simulink model "LoadFlow58BusNetwork_2024"  (R2024a)
settings: Solver=FixedStepDiscrete  StartTime=0.0  StopTime=4.5  FixedStep=75e-6  RelTol=1e-3  EnableMultiTasking=on
undefined symbols (not defined in the file): D1, D11, Delta
libraries: spsSeriesRLCBranchLib x41, spsLoadFlowBusLib x29, spsDistributedParametersLineLib x19, spsThreePhaseSeriesRLCLoadLib x15, spsThreePhaseTransformerTwoWindingsLib x13, spsThreePhaseParallelRLCLoadLib x11, spsThreePhaseVIMeasurementLib x11, spsSynchronousMachinepuStandardLib x7, spsExcitationSystemLib x7, spsHydraulicTurbineandGovernorLib x7, spsGenericPowerSystemStabilizerLib x7, spsMultiBandPowerSystemStabilizerLib x7
(part 3 of 5)

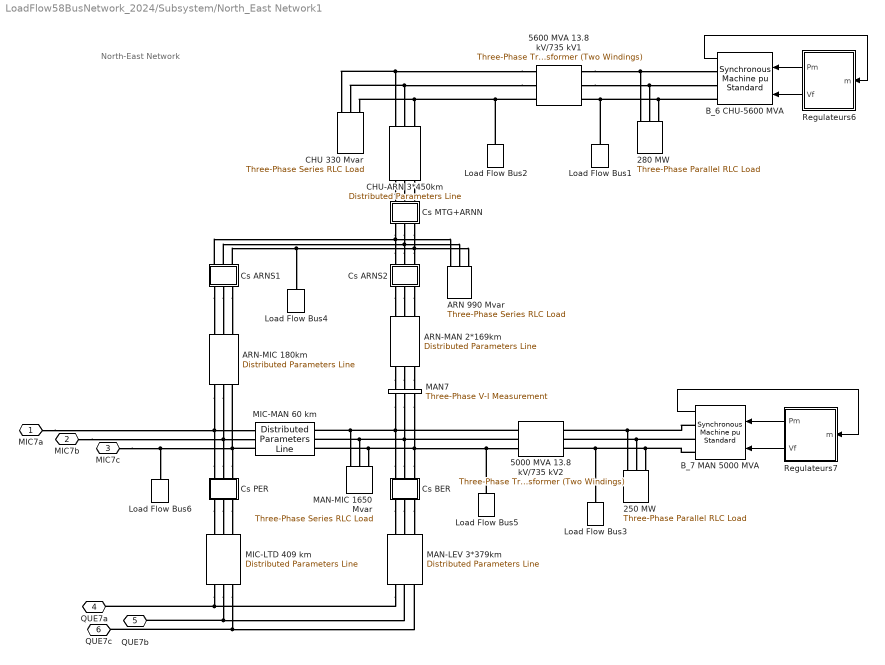
== system LoadFlow58BusNetwork_2024/Subsystem/North_East Network1 ==
  note: North-East Network
  250 MW : spsThreePhaseParallelRLCLoadLib/Three-Phase Parallel RLC Load  LConnTagsString=A|B|C  Configuration=Y (grounded)  NominalVoltage=(13800)*1  Vabc=[1e3 1e3 1e3]  Vabcp=[1e3 1e3 1e3]  NominalFrequency=60  UnbalancedPower=off  ActivePower=250000000  InductivePower=0  CapacitivePower=0  Pabc=[10e3 9e3 11e3]  QLabc=[100 90 110]  QCabc=[100 90 110]  Pabcp=[10e3 9e3 11e3]  QLabcp=[100 90 110]  QCabcp=[100 90 110]  Measurements=None  LoadType=constant PQ
  280 MW : spsThreePhaseParallelRLCLoadLib/Three-Phase Parallel RLC Load  LConnTagsString=A|B|C  Configuration=Y (grounded)  NominalVoltage=(13800)*1  Vabc=[1e3 1e3 1e3]  Vabcp=[1e3 1e3 1e3]  NominalFrequency=60  UnbalancedPower=off  ActivePower=280000000  InductivePower=0  CapacitivePower=0  Pabc=[10e3 9e3 11e3]  QLabc=[100 90 110]  QCabc=[100 90 110]  Pabcp=[10e3 9e3 11e3]  QLabcp=[100 90 110]  QCabcp=[100 90 110]  Measurements=None  LoadType=constant PQ
  5000 MVA 13.8 kV/735 kV2 : spsThreePhaseTransformerTwoWindingsLib/Three-Phase Transformer (Two Windings)  Winding1Connection=Delta (D1)  Winding2Connection=Yg  CoreType=Three single-phase transformers  SetSaturation=off  Hysteresis=off  DataFile='basic_model'  SetInitialFlux=off  Measurements=None  UNITS=pu  NominalPower=[ 5000e6 60 ]  Winding1="[ 13.8e3 0.002  0.0]"  Winding2=[ 735e3 0.002 0.12]  Rm=500  Lm=500  L0=0.5  Saturation="[ 0,0  ;  0.005,1.2  ;  1.0,1.4 ]"  InitialFluxes=[ 0.8 , -0.8 , 0.7 ]  BreakLoop=off  DiscreteSolver=Trapezoidal iterative  DataType=off  TransfoNumber=0
  5600 MVA 13.8 kV/735 kV1 : spsThreePhaseTransformerTwoWindingsLib/Three-Phase Transformer (Two Windings)  Winding1Connection=Delta (D1)  Winding2Connection=Yg  CoreType=Three single-phase transformers  SetSaturation=off  Hysteresis=off  DataFile='basic_model'  SetInitialFlux=off  Measurements=None  UNITS=pu  NominalPower=[ 5600e6 60 ]  Winding1="[ 13.8e3 0.002  0.0]"  Winding2=[ 735e3 0.002 0.12]  Rm=500  Lm=500  L0=0.5  Saturation="[ 0,0  ;  0.005,1.2  ;  1.0,1.4 ]"  InitialFluxes=[ 0.8 , -0.8 , 0.7 ]  BreakLoop=off  DiscreteSolver=Trapezoidal iterative  DataType=off  TransfoNumber=0
  ARN 990 Mvar : spsThreePhaseSeriesRLCLoadLib/Three-Phase Series RLC Load  LConnTagsString=A|B|C  Configuration=Y (grounded)  NominalVoltage=735e3  Vabc=[1e3 1e3 1e3]  Vabcp=[1e3 1e3 1e3]  NominalFrequency=60  UnbalancedPower=off  ActivePower=3300000  InductivePower=990e6  CapacitivePower=0  Pabc=[10e3 9e3 11e3]  QLabc=[100 90 110]  QCabc=[100 90 110]  Pabcp=[10e3 9e3 11e3]  QLabcp=[100 90 110]  QCabcp=[100 90 110]  Measurements=None  LoadType=constant Z
  ARN-MAN 2*169km : spsDistributedParametersLineLib/Distributed Parameters Line  Phases=3  Length=169  Frequency=60  Resistance="[0.01273  0.3864]/2"  Inductance="[0.9337e-3  4.1264e-3]/2"  Capacitance=[12.74e-9 7.751e-9]*2  x1=[-0.000975 1.60994599123016e-09 347873.977312517 -681165.145140754;-0.0009 1.53689774042001e-09 366991.883229411 -671058.367402052;-0.000825 1.46262091707149e-09 385816.421450015 -660415.155871986;-0.00075 1.38717489694071e-09 404332.543926502 -649244.018571007;-0.000675 1.31061999042181e-09 422525.449153869 -637553.885535348;-0.0006 1.23301739433572e-09 440380.594002039 -625354.101678494;-0.000525 1.1544291430104e-09 457883.705341412 -612654.419320997;-0.00045 1.07491805869151e-09 475020.791452591 -599464.990394622;-0.000375 9.94547701323305e-10 491778.153211145 -585796.358327047;-0.0003 9.13382317739751e-10 508142.39503848 -571659.449613611;-0.000225 8.31486790306614e-10 524100.43561006 -557065.565082836;-0.00015 7.4892658505548e-10 539639.51831242 -542026.370862723;-7.5e-05 6.65767699351214e-10 554747.221440602 -526553.889055024]  x2=[-0.000975 1.45072483719961e-09 232985.418240267 -689450.364518849;-0.0009 1.40774718437802e-09 252383.458947605 -682588.200672037;-0.000825 1.36364419999649e-09 271579.748179457 -675180.386261559;-0.00075 1.31845113930594e-09 290558.940715924 -667232.842980908;-0.000675 1.2722041289476e-09 309305.864880883 -658751.923974585;-0.0006 1.22494013807397e-09 327805.534669995 -649744.408759478;-0.000525 1.17669694879617e-09 346043.161730285 -640217.497805431;-0.00045 1.12751312598156e-09 364004.167181725 -630178.806779295;-0.000375 1.07742798642558e-09 381674.193271371 -619636.360457079;-0.0003 1.02648156742245e-09 399039.114850727 -608598.586309068;-0.000225 9.7471459476002e-10 416085.050667174 -597074.307763032;-0.00015 9.2216845016417e-10 432798.374460433 -585072.737150913;-7.5e-05 8.68885138218909e-10 449165.725855185 -572603.468344629]  x3=[-0.000975 -3.46324088240297e-12 1583.75858462542 -1421.24992657593;-0.0009 -3.61811610296408e-12 1623.30400424489 -1375.90902523653;-0.000825 -3.7700990568715e-12 1661.55177948074 -1329.46824327446;-0.00075 -3.91906825127732e-12 1698.47133564667 -1281.96470474027;-0.000675 -4.06490460248682e-12 1734.03315981437 -1233.43638323582;-0.0006 -4.20749153115222e-12 1768.20882440571 -1183.92207155882;-0.000525 -4.34671505546439e-12 1800.97100991732 -1133.46135069244;-0.00045 -4.4824638822682e-12 1832.29352675939 -1082.09455816485;-0.000375 -4.61462949602852e-12 1862.15133619119 -1029.86275580407;-0.0003 -4.74310624557591e-12 1890.52057033672 -976.807696913729;-0.000225 -4.86779142856255e-12 1917.37855126425 -922.971792896131;-0.00015 -4.9885853735609e-12 1942.70380911478 -868.398079349235;-7.5e-05 -5.10539151973954e-12 1966.47609926466 -813.130181664643]  x4=[-0.000975 1.11781487123881e-11 1569.30174481155 -9115.59279820464;-0.0009 1.10714227902124e-11 1826.37892658973 -9067.58416140609;-0.000825 1.09558465420566e-11 2081.99612899853 -9012.3270365676;-0.00075 1.08315123578052e-11 2335.94901555742 -8949.86559538931;-0.000675 1.06985196283027e-11 2588.03458021449 -8880.2497685916;-0.0006 1.05569746659022e-11 2838.0513096264 -8803.53520600126;-0.000525 1.04069906194808e-11 3085.79934424503 -8719.78323206585;-0.00045 1.02486873839906e-11 3331.08063808218 -8629.06079683187;-0.000375 1.00821915046157e-11 3573.6991170245 -8531.44042242597;-0.0003 9.90763607561482e-12 3813.46083557209 -8427.0001450818;-0.000225 9.72516063392696e-12 4050.17413187564 -8315.82345275907;-0.00015 9.53491104762829e-12 4283.64978094791 -8197.99921840458;-7.5e-05 9.33703939932717e-12 4513.70114592732 -8073.62162890849]  x5=0.000955765248222805  V1=ones(3,3)  V2=ones(3,3)  I1=ones(3,3)  I2=ones(3,3)  nHarmo=1  Measurements=None  Decoupling=on  VsMag0=[624500.542746141 624501.904306222 624500.043261921]  VrMag0=[594207.380493472 594208.10130569 594207.286862311]  VsAngle0=[18.1135948354222 -101.886530201489 138.113424134252]  VrAngle0=[9.73160889879769 -110.268441654031 129.731523430554]  IsMag0=[1744.35611857441 1744.39210598369 1744.37536737747]  IrMag0=[7582.44376493555 7582.43378992705 7582.40838117062]  IsAngle0=[39.1559168024775 -80.8440356055341 159.154916919463]  IrAngle0=[0.828149284034121 -119.172115933986 120.828081951988]
      settings: AttributesFormatString=\n  LibrarySourceBlock=sps_lib/Power Grid Elements/Distributed Parameters Line
  ARN-MIC 180km : spsDistributedParametersLineLib/Distributed Parameters Line  Phases=3  Length=180  Frequency=60  Resistance="[0.01273  0.3864]"  Inductance="[0.9337e-3  4.1264e-3]"  Capacitance=[12.74e-9 7.751e-9]  x1=[-0.00105 1.19354121063199e-09 336203.730988114 -674396.627297907;-0.000975 1.12512510468791e-09 355134.952563332 -664622.476598179;-0.0009 1.05580959095014e-09 373782.284691218 -654317.036859723;-0.000825 9.85650079179792e-10 392130.820979783 -643488.546093388;-0.00075 9.14702653817098e-10 410165.893889859 -632145.660429011;-0.000675 8.43024029148362e-10 427873.086460108 -620297.44719584;-0.0006 7.70671503969425e-10 445238.243831719 -607953.37767425;-0.000525 6.97702915781885e-10 462247.484563584 -595123.319524545;-0.00045 6.24176594558681e-10 478887.211728913 -581817.528898905;-0.000375 5.5015131611601e-10 495144.123784406 -568046.64224277;-0.0003 4.75686255128832e-10 511005.225203304 -553821.667792231;-0.000225 4.00840937827548e-10 526457.836863818 -539153.976774214;-0.00015 3.25675194413637e-10 541489.606184617 -524055.294316497;-7.5e-05 2.50249111232309e-10 556088.516999301 -508537.690074818]  x2=[-0.00105 4.52654920431781e-09 192165.578486817 -719334.039084965;-0.000975 4.47031749550698e-09 212424.764832674 -713613.931123342;-0.0009 4.41051228328839e-09 232514.142071731 -707323.371103839;-0.000825 4.34718137503364e-09 252417.651063202 -700467.387603885;-0.00075 4.2803753965018e-09 272119.381246533 -693051.461191792;-0.000675 4.21014775136993e-09 291603.583360062 -685081.520045664;-0.0006 4.13655457854304e-09 310854.682030736 -676563.935214511;-0.000525 4.05965470727746e-09 329857.288224832 -667505.515525323;-0.00045 3.97950961015369e-09 348596.211549706 -657913.502140201;-0.000375 3.8961833539361e-09 367056.472396769 -647795.562767882;-0.0003 3.80974254835898e-09 385223.31391595 -637159.785534291;-0.000225 3.72025629287972e-09 403082.213812101 -626014.672517016;-0.00015 3.62779612144176e-09 420618.895953895 -614369.132948876;-7.5e-05 3.53243594529146e-09 437819.341785948 -602232.476096019]  x3=[-0.00105 3.53596874152127e-12 149.00166074942 -364.540935538888;-0.000975 3.79801966073249e-12 159.247423691846 -360.18329187299;-0.0009 4.05703450113857e-12 169.365886680341 -355.537723194559;-0.000825 4.31280621023915e-12 179.348961170408 -350.607943100115;-0.00075 4.56513032804341e-12 189.188666845046 -345.397892380438;-0.000675 4.81380515051227e-12 198.877137994092 -339.911735870358;-0.0006 5.05863189079749e-12 208.406629801948 -334.153859119447;-0.000525 5.29941483814888e-12 217.769524538669 -328.128864886281;-0.00045 5.53596151436242e-12 226.958337649459 -321.841569459065;-0.000375 5.76808282764443e-12 235.96572373771 -315.296998805564;-0.0003 5.99559322376864e-12 244.784482436803 -308.500384555424;-0.000225 6.21831083440543e-12 253.407564165964 -301.457159818085;-0.00015 6.43605762250454e-12 261.828075765596 -294.172954839637;-7.5e-05 6.6486595246152e-12 270.039286007565 -286.653592502086]  x4=[-0.00105 4.83329412277315e-12 1187.65933351918 -4979.46515427106;-0.000975 4.45670929323629e-12 1327.95758028639 -4943.89904376734;-0.0009 4.07656183848036e-12 1467.19427808235 -4904.38085601222;-0.000825 3.69315564256423e-12 1605.25812322123 -4860.94218124035;-0.00075 3.30679719453461e-12 1742.03874957769 -4813.61774366371;-0.000675 2.91779534342338e-12 1877.42681681182 -4762.4453737136;-0.0006 2.52646105135838e-12 2011.31409777419 -4707.46597779961;-0.000525 2.13310714498507e-12 2143.59356502093 -4648.7235056096;-0.00045 1.7380480653977e-12 2274.15947636987 -4586.26491497707;-0.000375 1.34159961677987e-12 2402.90745942922 -4520.14013434371;-0.0003 9.44078713955551e-13 2529.73459503121 -4450.40202284742;-0.000225 5.45803129052187e-13 2654.53949950417 -4377.1063280675;-0.00015 1.47091237478525e-13 2777.22240571704 -4300.31164146089;-7.5e-05 -2.51738236579805e-13 2897.68524283171 -4220.07935152508]  x5=0.00101797482059234  V1=ones(3,3)  V2=ones(3,3)  I1=ones(3,3)  I2=ones(3,3)  nHarmo=1  Measurements=None  Decoupling=on  VsMag0=[615273.936100311 615275.237959029 615273.425867059]  VrMag0=[607930.23167611 607930.976808519 607930.152146887]  VsAngle0=[19.1774103741909 -100.822714483793 139.177242954885]  VrAngle0=[7.63692875074935 -112.363120449623 127.636843332422]  IsMag0=[322.896150602406 322.910343515381 322.909058922126]  IrMag0=[4197.50413399086 4197.49907033608 4197.48826872802]  IsAngle0=[14.9112658694316 -105.087543385488 134.909680310748]  IrAngle0=[6.09512812442721 -113.905082032175 126.09508290497]
      settings: AttributesFormatString=\n  LibrarySourceBlock=sps_lib/Power Grid Elements/Distributed Parameters Line
  "B_6 CHU-5600 MVA " : spsSynchronousMachinepuStandardLib/Synchronous Machine pu Standard  PresetModel=No  MechanicalLoad=Mechanical power Pm  ShowDetailedParameters=on  RotorType=Salient-pole  Units=per unit standard parameters  MeasurementBus=off  NominalParameters="[ 5600E6  13800   60 ]"  Reactances1=[ 31 32 33 34 35 36 37 ]  Reactances2=[ 1.305, 0.296, 0.252, 0.474, 0.243, 0.18 ]  dAxisTimeConstants=Short-circuit  qAxisTimeConstants=Open-circuit  TimeConstants1=[]  TimeConstants2=[]  TimeConstants3=[]  TimeConstants4=[]  TimeConstants5=[ 1.01, 0.053, 0.1 ]  TimeConstants6=[]  TimeConstants7=[]  TimeConstants8=[]  StatorResistance=2.8544e-3  Mechanical="[ 4.0 0  32]"  PolePairs=32  InitialConditions=[0 -61.7964 0.894782 0.894782 0.894782 8.48442 -111.516 128.484 1.31361]  SetSaturation=off  Saturation=[0.6404,0.7127,0.8441,0.9214,0.9956,1.082,1.19,1.316,1.457;0.7,0.7698,0.8872,0.9466,0.9969,1.046,1.1,1.151,1.201]  LoadFlowParameters=[1 5000000000 0 0 0]  TsPowergui=0  TsBlock=-1  IterativeModel=Trapezoidal non iterative  IterativeDiscreteModel=Trapezoidal non iterative  BusType=PV  Pref=5000000000  Qref=0  Qmin=-Inf  Qmax=Inf  PLF=0  QLF=0
  B_7 MAN 5000 MVA : spsSynchronousMachinepuStandardLib/Synchronous Machine pu Standard  PresetModel=No  MechanicalLoad=Mechanical power Pm  ShowDetailedParameters=on  RotorType=Salient-pole  Units=per unit standard parameters  MeasurementBus=off  NominalParameters="[ 5000E6  13800   60 ]"  Reactances1=[ 31 32 33 34 35 36 37 ]  Reactances2=[ 1.305, 0.296, 0.252, 0.474, 0.243, 0.18 ]  dAxisTimeConstants=Short-circuit  qAxisTimeConstants=Open-circuit  TimeConstants1=[]  TimeConstants2=[]  TimeConstants3=[]  TimeConstants4=[]  TimeConstants5=[ 1.01, 0.053, 0.1 ]  TimeConstants6=[]  TimeConstants7=[]  TimeConstants8=[]  StatorResistance=2.8544e-3  Mechanical="[ 3.7 0  32]"  PolePairs=32  InitialConditions=[0 -81.9543 0.907703 0.907703 0.907703 -8.76021 -128.76 111.24 1.25655]  SetSaturation=off  Saturation=[0.6404,0.7127,0.8441,0.9214,0.9956,1.082,1.19,1.316,1.457;0.7,0.7698,0.8872,0.9466,0.9969,1.046,1.1,1.151,1.201]  LoadFlowParameters=[1 4500000000 0 0 0]  TsPowergui=0  TsBlock=-1  IterativeModel=Trapezoidal non iterative  IterativeDiscreteModel=Trapezoidal non iterative  BusType=PV  Pref=4500000000  Qref=0  Qmin=-Inf  Qmax=Inf  PLF=0  QLF=0
  CHU 330 Mvar : spsThreePhaseSeriesRLCLoadLib/Three-Phase Series RLC Load  LConnTagsString=A|B|C  Configuration=Y (grounded)  NominalVoltage=735e3  Vabc=[1e3 1e3 1e3]  Vabcp=[1e3 1e3 1e3]  NominalFrequency=60  UnbalancedPower=off  ActivePower=1100000  InductivePower=330e6  CapacitivePower=0  Pabc=[10e3 9e3 11e3]  QLabc=[100 90 110]  QCabc=[100 90 110]  Pabcp=[10e3 9e3 11e3]  QLabcp=[100 90 110]  QCabcp=[100 90 110]  Measurements=None  LoadType=constant Z
  CHU-ARN 3*450km : spsDistributedParametersLineLib/Distributed Parameters Line  Phases=3  Length=450  Frequency=60  Resistance="[0.01273  0.3864]/3"  Inductance="[0.9337e-3  4.1264e-3]/3"  Capacitance=[12.74e-9 7.751e-9]*3  x1=[-0.00255 1.80867377993606e-09 0 0;-0.002475 1.72308488593625e-09 0 0;-0.0024 1.6361185842427e-09 0 0;-0.002325 1.54784439438636e-09 0 0;-0.00225 1.45833288140396e-09 0 0;-0.002175 1.36765559942941e-09 0 0;-0.0021 1.2758850344945e-09 0 0;-0.002025 1.18309454658472e-09 0 0;-0.00195 1.08935831099635e-09 0 0;-0.001875 9.94751259041912e-10 0 0;-0.0018 8.993490181512e-10 0 0;-0.001725 8.03227851415879e-10 0 0;-0.00165 7.06464596625934e-10 0 0;-0.001575 6.09136604846718e-10 336692.129653521 -649852.524072729;-0.0015 5.1132167858569e-10 354929.318551966 -640074.408280399;-0.001425 4.13098009598284e-10 372882.782383762 -629784.626799556;-0.00135 3.14544116382617e-10 390538.169424619 -618991.405124078;-0.001275 2.15738781413e-10 407881.366228272 -607703.37119023;-0.0012 1.16760988162435e-10 424898.508908555 -595929.548479625;-0.001125 1.76898579644369e-11 441575.994221983 -583679.348805994;-0.00105 -8.13954132353542e-11 457900.490441969 -570962.564791521;-0.000975 -1.80415618187197e-10 473858.948016008 -557789.362038774;-0.0009 -2.79291601654312e-10 489438.609997288 -544170.271004476;-0.000825 -3.7794432368837e-10 504627.022242398 -530116.178581621;-0.00075 -4.76294922812813e-10 519412.04336698 -515638.319396658;-0.000675 -5.74264779063516e-10 533781.854451365 -500748.266828701;-0.0006 -6.71775576836382e-10 547724.968488438 -485457.923757945;-0.000525 -7.68749367491635e-10 561230.239566175 -469779.513050693;-0.00045 -8.65108631664776e-10 574286.871777512 -453725.567788576;-0.000375 -9.60776341234369e-10 586884.427850435 -437308.921249803;-0.0003 -1.05567602089715e-09 599012.837491367 -420542.696650433;-0.000225 -1.14973180930121e-09 610662.405435212 -403440.29665388;-0.00015 -1.24286851968841e-09 621823.8191956 -386015.392657025;-7.5e-05 -1.33501169999749e-09 632488.156509147 -368281.913861514]  x2=[-0.00255 2.59530396061635e-09 0 0;-0.002475 2.56712725861336e-09 0 0;-0.0024 2.53689843435821e-09 0 0;-0.002325 2.50464165231048e-09 0 0;-0.00225 2.47038269804819e-09 0 0;-0.002175 2.43414895765521e-09 0 0;-0.0021 2.39596939582921e-09 0 0;-0.002025 2.35587453272774e-09 0 0;-0.00195 2.3138964195709e-09 0 0;-0.001875 2.27006861302005e-09 0 0;-0.0018 2.22442614835317e-09 0 0;-0.001725 2.17700551145816e-09 0 0;-0.00165 2.12784460966659e-09 0 0;-0.001575 2.07698274145117e-09 24661.2186379731 -733238.396736884;-0.0015 2.02446056501113e-09 45380.4401577959 -732248.159297742;-0.001425 1.97032006577071e-09 66063.3852481006 -730672.57388383;-0.00135 1.91460452281662e-09 86693.5202790416 -728512.899994021;-0.001275 1.85735847430142e-09 107254.353836327 -725770.864038578;-0.0012 1.79862768184041e-09 127729.449904202 -722448.657959089;-0.001125 1.73845909393045e-09 148102.44100415 -718548.937476262;-0.00105 1.67690080842013e-09 168357.041278802 -714074.819966984;-0.000975 1.61400203406099e-09 188477.059510606 -709029.881972336;-0.0009 1.54981305117089e-09 208446.412064832 -703418.15633856;-0.000825 1.48438517144061e-09 228249.135746591 -697244.128993266;-0.00075 1.41777069691614e-09 247869.400561563 -690512.735359448;-0.000675 1.35002287818918e-09 267291.522370255 -683229.356410182;-0.0006 1.28119587182943e-09 286499.975425661 -675399.814367161;-0.000525 1.2113446970927e-09 305479.404784309 -667030.3680465;-0.00045 1.1405251919393e-09 324214.638580764 -658127.707855528;-0.000375 1.06879396839809e-09 342690.700155788 -648698.950444589;-0.0003 9.96208367311644e-10 360892.82002845 -638751.633018091;-0.000225 9.22826412498863e-10 378806.447702628 -628293.707309386;-0.00015 8.48706764371648e-10 396417.263298445 -617333.533224274;-7.5e-05 7.73908673042644e-10 413711.188999368 -605879.872158222]  x3=[-0.00255 4.24136020094849e-12 0 0;-0.002475 4.2220551602755e-12 0 0;-0.0024 4.199375073307e-12 0 0;-0.002325 4.17333807015748e-12 0 0;-0.00225 4.1439649644089e-12 0 0;-0.002175 4.11127923647256e-12 0 0;-0.0021 4.07530701481927e-12 0 0;-0.002025 4.03607705509262e-12 0 0;-0.00195 3.99362071712217e-12 0 0;-0.001875 3.94797193985491e-12 0 0;-0.0018 3.89916721422492e-12 0 0;-0.001725 3.84724555398313e-12 0 0;-0.00165 3.79224846451033e-12 0 0;-0.001575 3.73421990963834e-12 -336.540930618498 -2064.60581280805;-0.0015 3.67320627650607e-12 -278.039507495715 -2073.29664773843;-0.001425 3.6092563384783e-12 -219.315823844787 -2080.33012105111;-0.00135 3.54242121615703e-12 -160.416822479922 -2085.70061029514;-0.001275 3.47275433651642e-12 -101.389586361627 -2089.40382238359;-0.0012 3.40031139019412e-12 -42.2813009593069 -2091.43679702537;-0.001125 3.32515028697301e-12 16.8607834680746 -2091.79790909167;-0.00105 3.247331109489e-12 75.9893896431304 -2090.48686991503;-0.000975 3.16691606520189e-12 135.057251062782 -2087.50472752009;-0.0009 3.08396943666771e-12 194.017149782379 -2082.85386578587;-0.000825 2.99855753015217e-12 252.821954161003 -2076.53800254008;-0.00075 2.91074862262649e-12 311.424656537775 -2068.56218658714;-0.000675 2.82061290718783e-12 369.778410809068 -2058.93279367232;-0.0006 2.72822243694799e-12 427.83656987656 -2047.65752138496;-0.000525 2.63365106743526e-12 485.552722936212 -2034.74538300522;-0.00045 2.53697439755543e-12 542.880732578354 -2020.20670029895;-0.000375 2.43826970915921e-12 599.774771669227 -2004.05309526666;-0.0003 2.33761590526426e-12 656.189359984489 -1986.29748085305;-0.000225 2.23509344698136e-12 712.079400565414 -1966.95405062462;-0.00015 2.13078428919503e-12 767.400215768706 -1946.03826742353;-7.5e-05 2.02477181505001e-12 822.10758298113 -1923.56685100685]  x4=[-0.00255 1.92507826273785e-11 0 0;-0.002475 1.90857971627026e-11 0 0;-0.0024 1.89055548037973e-11 0 0;-0.002325 1.87101996336465e-11 0 0;-0.00225 1.84998878161842e-11 0 0;-0.002175 1.82747874714595e-11 0 0;-0.0021 1.80350785412437e-11 0 0;-0.002025 1.7780952645188e-11 0 0;-0.00195 1.75126129276454e-11 0 0;-0.001875 1.72302738952804e-11 0 0;-0.0018 1.69341612455956e-11 0 0;-0.001725 1.66245116865124e-11 0 0;-0.00165 1.63015727471505e-11 0 0;-0.001575 1.5965602579957e-11 -291.74302430487 -14207.2379327614;-0.0015 1.5616869754343e-11 110.022151991721 -14209.8063832457;-0.001425 1.52556530419935e-11 511.699378263407 -14201.0157319245;-0.00135 1.48822411940216e-11 912.967559881373 -14180.8730059101;-0.001275 1.44969327101451e-11 1313.50592920084 -14149.3943069894;-0.0012 1.41000356000706e-11 1712.99430197782 -14106.6047987527;-0.001125 1.36918671372751e-11 2111.11333331949 -14052.5386864782;-0.00105 1.32727536053828e-11 2507.54477296362 -13987.2391897887;-0.000975 1.28430300373382e-11 2901.97171968297 -13910.7585081029;-0.0009 1.24030399475867e-11 3294.07887461125 -13823.1577789074;-0.000825 1.1953135057474e-11 3683.55279328827 -13724.5070288849;-0.00075 1.14936750140855e-11 4070.08213622259 -13614.8851179355;-0.000675 1.10250271027498e-11 4453.35791777155 -13494.3796761375;-0.0006 1.05475659534367e-11 4833.0737531397 -13363.0870336974;-0.000525 1.00616732412837e-11 5208.92610329811 -13221.1121439446;-0.00045 9.56773738149033e-12 5580.61451762878 -13068.5684994337;-0.000375 9.06615321882548e-12 5947.84187410032 -12905.5780412202;-0.0003 8.55732171199431e-12 6310.31461678274 -12732.2710613825;-0.000225 8.04164961311797e-12 6667.74299051156 -12548.7860988686;-0.00015 7.51954914258228e-12 7019.84127251364 -12355.2698287502;-7.5e-05 6.99143765951497e-12 7366.32800080966 -12151.8769449726]  x5=0.00254493705148084  V1=ones(3,3)  V2=ones(3,3)  I1=ones(3,3)  I2=ones(3,3)  nHarmo=1  Measurements=None  Decoupling=on  VsMag0=[597589.636778606 597591.191030923 597588.179734111]  VrMag0=[599025.218159244 599025.681050624 599025.14641932]  VsAngle0=[31.4089201475954 -88.5913271983218 151.408667420084]  VrAngle0=[5.94632207994268 -114.053711405456 125.94626699413]  IsMag0=[1726.1254830947 1726.16866029042 1726.16794416601]  IrMag0=[11726.0675753704 11726.0492062867 11726.0164561755]  IsAngle0=[-5.23898774451376 -125.238187761859 114.760171100737]  IrAngle0=[2.8437567880639 -117.156479810909 122.843716218955]
      settings: AttributesFormatString=\n  LibrarySourceBlock=sps_lib/Power Grid Elements/Distributed Parameters Line
  "Cs ARNS1 " : Subsystem  mask{Xc=25}
      mask prompts: Xc "Condensator Reactance at  60Hz  (ohm):"
      mask help: Series Compensation
      mask init:
      | Cs=1/Xc/(2*pi*60);
      mask Display: disp('Cs')
  Cs ARNS2 : Subsystem  mask{Xc=25/2}
      mask prompts: Xc "Condensator Reactance at  60Hz  (ohm):"
      mask help: Series Compensation
      mask init:
      | Cs=1/Xc/(2*pi*60);
      mask Display: disp('Cs')
  Cs BER : Subsystem  mask{Xc=22/3}
      mask prompts: Xc "Condensator Reactance at  60Hz  (ohm):"
      mask help: Series Compensation
      mask init:
      | Cs=1/Xc/(2*pi*60);
      mask Display: disp('Cs')
  "Cs MTG+ARNN " : Subsystem  mask{Xc=(30+25)/3}
      mask prompts: Xc "Condensator Reactance at  60Hz  (ohm):"
      mask help: Series Compensation
      mask init:
      | Cs=1/Xc/(2*pi*60);
      mask Display: disp('Cs')
  "Cs PER " : Subsystem  mask{Xc=22}
      mask prompts: Xc "Condensator Reactance at  60Hz  (ohm):"
      mask help: Series Compensation
      mask init:
      | Cs=1/Xc/(2*pi*60);
      mask Display: disp('Cs')
  Load Flow Bus1 : spsLoadFlowBusLib/Load Flow Bus  LConnTagsString=a  Phases=single  Connectors=on one side  ID=CHU_13.8  Vbase=13.8e3  Vref=1  Vangle=0  VLF=1  VLFb=1  VLFc=1  angleLF=4.726  angleLFb=0  angleLFc=0
      settings: AttributesFormatString=%<ID>\n%<Vbase>V\n%<VLF>pu\n%<angleLF>deg.
  Load Flow Bus2 : spsLoadFlowBusLib/Load Flow Bus  LConnTagsString=a  Phases=single  Connectors=on one side  ID=CHU7  Vbase=735e3  Vref=1  Vangle=0  VLF=1.009  VLFb=1  VLFc=1  angleLF=28.97  angleLFb=0  angleLFc=0
      settings: AttributesFormatString=%<ID>\n%<Vbase>V\n%<VLF>pu\n%<angleLF>deg.
  Load Flow Bus3 : spsLoadFlowBusLib/Load Flow Bus  LConnTagsString=a  Phases=single  Connectors=on one side  ID=MAN_13.8  Vbase=13.8e3  Vref=1  Vangle=0  VLF=1  VLFb=1  VLFc=1  angleLF=-16.23  angleLFb=0  angleLFc=0
      settings: AttributesFormatString=%<ID>\n%<Vbase>V\n%<VLF>pu\n%<angleLF>deg.
  Load Flow Bus4 : spsLoadFlowBusLib/Load Flow Bus  LConnTagsString=a  Phases=single  Connectors=on one side  ID=ARN7  Vbase=735e3  Vref=1  Vangle=0  VLF=1.054  VLFb=1  VLFc=1  angleLF=12.72  angleLFb=0  angleLFc=0
      settings: AttributesFormatString=%<ID>\n%<Vbase>V\n%<VLF>pu\n%<angleLF>deg.
  Load Flow Bus5 : spsLoadFlowBusLib/Load Flow Bus  LConnTagsString=a  Phases=single  Connectors=on one side  ID=MAN7  Vbase=735e3  Vref=1  Vangle=0  VLF=1.016  VLFb=1  VLFc=1  angleLF=7.996  angleLFb=0  angleLFc=0
      settings: AttributesFormatString=%<ID>\n%<Vbase>V\n%<VLF>pu\n%<angleLF>deg.
  Load Flow Bus6 : spsLoadFlowBusLib/Load Flow Bus  LConnTagsString=a  Phases=single  Connectors=on one side  ID=MIC7  Vbase=735e3  Vref=1  Vangle=0  VLF=1.041  VLFb=1  VLFc=1  angleLF=5.981  angleLFb=0  angleLFc=0
      settings: AttributesFormatString=%<ID>\n%<Vbase>V\n%<VLF>pu\n%<angleLF>deg.
  MAN-LEV 3*379km : spsDistributedParametersLineLib/Distributed Parameters Line  Phases=3  Length=379  Frequency=60  Resistance="[0.01273  0.3864]/3"  Inductance="[0.9337e-3  4.1264e-3]/3"  Capacitance=[12.74e-9 7.751e-9]*3  x1=[-0.002175 3.20011367306785e-09 -30838.3336726537 -721772.96842408;-0.0021 3.15830158139619e-09 -10421.0500053442 -722356.328523331;-0.002025 3.11396479176399e-09 10004.5640898923 -722362.248025983;-0.00195 3.06713874632251e-09 30422.1806896704 -721790.722200075;-0.001875 3.01786087709602e-09 50815.47826368 -720642.20791461;-0.0018 2.96617057605919e-09 71168.1547218684 -718917.623274333;-0.001725 2.9121091636478e-09 91463.9404460816 -716618.346885819;-0.00165 2.85571985572775e-09 111686.611295747 -713746.216755433;-0.001575 2.79704772904902e-09 131820.001577206 -710303.528820056;-0.0015 2.73613968521194e-09 151848.016966317 -706293.035111749;-0.001425 2.67304441317485e-09 171754.647374018 -701717.941557819;-0.00135 2.60781235033282e-09 191523.979744542 -696581.905418053;-0.001275 2.5404956421988e-09 211140.210776074 -690889.032361155;-0.0012 2.47114810071929e-09 230587.659553665 -684643.873182745;-0.001125 2.3998251612579e-09 249850.780084318 -677851.420167516;-0.00105 2.32658383828115e-09 268914.173724217 -670517.103098478;-0.000975 2.25148267978202e-09 287762.601488166 -662646.78491648;-0.0009 2.1745817204775e-09 306380.9962314 -654246.757033455;-0.000825 2.09594243381785e-09 324754.474694034 -645323.734303169;-0.00075 2.0156276828456e-09 342868.349398507 -635884.849653465;-0.000675 1.93370166994382e-09 360708.140390532 -625937.648384312;-0.0006 1.85022988551372e-09 378259.58681415 -615490.082136208;-0.000525 1.7652790556226e-09 395508.658311633 -604550.502533759;-0.00045 1.6789170886641e-09 412441.566239148 -593127.654509517;-0.000375 1.5912130210732e-09 429044.774689179 -581230.669313417;-0.0003 1.50223696213964e-09 445305.011310928 -568869.057213396;-0.000225 1.41206003796354e-09 461209.27792003 -556052.699893027;-0.00015 1.32075433459834e-09 476744.860889102 -542791.842552255;-7.5e-05 1.22839284042627e-09 491899.34131082 -529097.08571754]  x2=[-0.002175 1.38351872909083e-08 -379192.175232135 -624794.196144335;-0.0021 1.38990649351923e-08 -361377.32073441 -635264.451513569;-0.002025 1.39518318796298e-08 -343273.586735748 -645226.886200136;-0.00195 1.3993445943133e-08 -324895.445084111 -654673.536386177;-0.001875 1.40238738600562e-08 -306257.586984741 -663596.850564071;-0.0018 1.40430913067881e-08 -287374.911256234 -671989.695572997;-0.001725 1.40510829211958e-08 -268262.512420652 -679845.362301069;-0.00165 1.40478423149052e-08 -248935.668637195 -687157.5710485;-0.001575 1.40333720784072e-08 -229409.829489073 -693920.476547499;-0.0015 1.40076837789875e-08 -209700.603633346 -700128.672634885;-0.001425 1.39707979514796e-08 -189823.746323601 -705777.196573694;-0.00135 1.39227440818497e-08 -169795.146815445 -710861.533020316;-0.001275 1.38635605836259e-08 -149630.815664878 -715377.617633987;-0.0012 1.37932947671911e-08 -129346.871929697 -719321.840325766;-0.001125 1.37120028019639e-08 -108959.530284169 -722691.048144382;-0.00105 1.36197496714975e-08 -88485.0880572684 -725482.547796656;-0.000975 1.35166091215329e-08 -67939.9122048419 -727694.107800476;-0.0009 1.34026636010476e-08 -47340.4262261144 -729323.960268613;-0.000825 1.32780041963472e-08 -26703.0970349947 -730370.802321943;-0.00075 1.31427305582526e-08 -6044.42179667621 -730833.797130944;-0.000675 1.29969508224402e-08 14619.0852599438 -730712.574584651;-0.0006 1.28407815230003e-08 35270.9060434865 -730007.231586512;-0.000525 1.26743474992815e-08 55894.531804401 -728718.331976929;-0.00045 1.24977817960958e-08 76473.4763318061 -726846.906082527;-0.000375 1.23112255573648e-08 96991.2891323149 -724394.449892533;-0.0003 1.21148279132913e-08 117431.568580308 -721362.923862902;-0.000225 1.1908745861147e-08 137777.975029141 -717754.751349158;-0.00015 1.16931441397712e-08 158014.24387281 -713572.816669202;-7.5e-05 1.14681950978812e-08 178124.198547625 -708820.46279763]  x3=[-0.002175 6.58584377734838e-12 -359.273937221319 349.814819581325;-0.0021 8.15999498110593e-12 -369.020063583709 339.517457528038;-0.002025 9.7276232097277e-12 -378.471200953466 328.948690413994;-0.00195 1.12874753251933e-11 -387.619794235985 318.116966749918;-0.001875 1.2838304405588e-11 -396.458530185773 307.030945249974;-0.0018 1.43788707418736e-11 -404.980343252549 295.699487910128;-0.001725 1.59079428288922e-11 -413.178421229337 284.131652924001;-0.00165 1.74242983498131e-11 -421.046210698035 272.336687441887;-0.001575 1.89267251532338e-11 -428.577422268125 260.324020178722;-0.0015 2.04140222221557e-11 -435.766035604308 248.103253876918;-0.001425 2.18850006340581e-11 -442.606304239072 235.684157630072;-0.00135 2.33384845113055e-11 -449.092760166332 223.076659073705;-0.001275 2.47733119611253e-11 -455.220218212464 210.290836449261;-0.0012 2.61883360044078e-11 -460.98378018126 197.336910547718;-0.001125 2.75824254925833e-11 -466.378838769468 184.225236539239;-0.00105 2.89544660118453e-11 -471.401081249799 170.966295695411;-0.000975 3.03033607739956e-11 -476.046492918457 157.570687010676;-0.0009 3.16280314932002e-11 -480.311360304431 144.049118729657;-0.000825 3.29274192479542e-11 -484.192274137989 130.412399787151;-0.00075 3.42004853275678e-11 -487.686132075991 116.671431167632;-0.000675 3.54462120624955e-11 -490.790141181859 102.83719719117;-0.0006 3.66636036378457e-11 -493.501820158208 88.9207567327353;-0.000525 3.78516868894197e-11 -495.819001330353 74.9332343819018;-0.00045 3.90095120816446e-11 -497.73983237912 60.8858115500204;-0.000375 4.01361536667769e-11 -499.262777821557 46.78971753197;-0.0003 4.12307110247718e-11 -500.386620238381 32.6562205296313;-0.000225 4.22923091832245e-11 -501.110461247159 18.4966186442581;-0.00015 4.33200995168102e-11 -501.433722220462 4.32223084494839;-7.5e-05 4.43132604256619e-11 -501.356144748416 -9.85561207956639]  x4=[-0.002175 5.32822560666844e-11 -7842.63207577957 -13937.1348474411;-0.0021 5.25232661185771e-11 -7445.48599612257 -14153.2795346858;-0.002025 5.17222898751674e-11 -7042.38810888003 -14358.1103068229;-0.00195 5.08799676246092e-11 -6633.6606443354 -14551.4634252672;-0.001875 4.99969727064214e-11 -6219.6303329701 -14733.1843264942;-0.0018 4.90740109732314e-11 -5800.62814428016 -14903.1277455959;-0.001725 4.8111820226527e-11 -5376.98902220426 -15061.1578324032;-0.00165 4.7111169626869e-11 -4949.05161737471 -15207.1482600828;-0.001575 4.60728590790364e-11 -4517.15801640526 -15340.9823261204;-0.0015 4.49977185925944e-11 -4081.65346843233 -15462.5530456115;-0.001425 4.38866076183977e-11 -3642.88610912813 -15571.7632367828;-0.00135 4.27404143615584e-11 -3201.20668240631 -15668.5255986787;-0.001275 4.15600550714287e-11 -2756.96826004269 -15752.7627809474;-0.0012 4.03464733091651e-11 -2310.52595943501 -15824.4074456744;-0.001125 3.910063919346e-11 -1862.2366597276 -15883.4023212109;-0.00105 3.78235486250434e-11 -1412.45871652758 -15929.700247956;-0.000975 3.65162224905756e-11 -961.551675440905 -15963.2642160555;-0.0009 3.51797058465658e-11 -509.875984657118 -15984.0673949868;-0.000825 3.38150670839699e-11 -57.7927068125609 -15992.093155007;-0.00075 3.24233970741348e-11 394.336769637563 -15987.3350804463;-0.000675 3.10058082967734e-11 846.151019307595 -15969.7969748367;-0.0006 2.95634339506642e-11 1297.28886879934 -15939.4928578716;-0.000525 2.80974270477906e-11 1747.38968541855 -15896.4469541982;-0.00045 2.66089594916401e-11 2196.09366545919 -15840.6936740535;-0.000375 2.50992211404026e-11 2643.04212182502 -15772.2775857565;-0.0003 2.35694188558165e-11 3087.87777075857 -15691.2533800813;-0.000225 2.20207755384213e-11 3530.24501744829 -15597.6858265384;-0.00015 2.04545291499898e-11 3969.79024028562 -15491.6497215983;-7.5e-05 1.88719317239206e-11 4406.1620735447 -15373.2298289009]  x5=0.00214340253891386  V1=ones(3,3)  V2=ones(3,3)  I1=ones(3,3)  I2=ones(3,3)  nHarmo=1  Measurements=None  Decoupling=on  VsMag0=[589863.022608861 589863.802580087 589862.857709079]  VrMag0=[596743.737336323 596743.911083336 596743.706580344]  VsAngle0=[14.5334919446082 -105.466570291736 134.533395214791]  VrAngle0=[-14.273856882167 -134.273869923453 105.726122150021]  IsMag0=[413.109398328918 413.092934231415 413.107596304112]  IrMag0=[13174.467520531 13174.4678533388 13174.4493337438]  IsAngle0=[-117.256344753877 122.74468499819 2.74614766436527]  IrAngle0=[-12.3870102586423 -132.387102424573 107.612942404921]
      settings: AttributesFormatString=\n  LibrarySourceBlock=sps_lib/Power Grid Elements/Distributed Parameters Line
  MAN-MIC 1650 Mvar : spsThreePhaseSeriesRLCLoadLib/Three-Phase Series RLC Load  LConnTagsString=A|B|C  Configuration=Y (grounded)  NominalVoltage=735e3  Vabc=[1e3 1e3 1e3]  Vabcp=[1e3 1e3 1e3]  NominalFrequency=60  UnbalancedPower=off  ActivePower=5500000  InductivePower=1650e6  CapacitivePower=0  Pabc=[10e3 9e3 11e3]  QLabc=[100 90 110]  QCabc=[100 90 110]  Pabcp=[10e3 9e3 11e3]  QLabcp=[100 90 110]  QCabcp=[100 90 110]  Measurements=None  LoadType=constant Z
  MAN7 : spsThreePhaseVIMeasurementLib/Three-Phase V-I Measurement  VoltageMeasurement=no  SetLabelV=on  LabelV=Vabc_MAN7  Vpu=on  VpuLL=off  CurrentMeasurement=no  SetLabelI=on  LabelI=Iabc_MAN7  Ipu=on  Pbase=100e6  Vbase=735e3  OutputType=Magnitude  PhasorSimulation=off  PSBequivalent=0
  MIC-LTD 409 km : spsDistributedParametersLineLib/Distributed Parameters Line  Phases=3  Length=409  Frequency=60  Resistance="[0.01273  0.3864]"  Inductance="[0.9337e-3  4.1264e-3]"  Capacitance=[12.74e-9 7.751e-9]  x1=[-0.002325 4.55344961412385e-09 0 0;-0.00225 4.56222172896998e-09 0 0;-0.002175 4.5673468735703e-09 0 0;-0.0021 4.56882095096264e-09 0 0;-0.002025 4.56664278279209e-09 0 0;-0.00195 4.56081411025295e-09 0 0;-0.001875 4.55133959269686e-09 0 0;-0.0018 4.53822680390821e-09 0 0;-0.001725 4.52148622604971e-09 0 0;-0.00165 4.50113124128317e-09 0 0;-0.001575 4.47717812107196e-09 0 0;-0.0015 4.44964601317389e-09 0 0;-0.001425 4.41855692633476e-09 138503.934059085 -724390.238526683;-0.00135 4.3839357126949e-09 158927.516108443 -720185.156863818;-0.001275 4.34581004792278e-09 179224.053933097 -715404.370205759;-0.0012 4.30421040909147e-09 199377.322791257 -710051.700240211;-0.001125 4.25917005031577e-09 219371.212468153 -704131.425809646;-0.00105 4.21072497616932e-09 239189.740154295 -697648.279490861;-0.000975 4.15891391290319e-09 258817.063221882 -690607.443811828;-0.0009 4.10377827748859e-09 278237.491889164 -683014.54710886;-0.000825 4.04536214450888e-09 297435.501762606 -674875.659027406;-0.00075 3.98371221092697e-09 316395.746246855 -666197.285670069;-0.000675 3.91887775875648e-09 335103.068812571 -656986.364395728;-0.0006 3.85091061566648e-09 353542.515112327 -647250.258273917;-0.000525 3.77986511355123e-09 371699.344934885 -636996.750198904;-0.00045 3.70579804509808e-09 389559.043988292 -626234.036668158;-0.000375 3.62876861838829e-09 407107.335502388 -614970.721230202;-0.0003 3.54883840956699e-09 424330.191641435 -603215.807607062;-0.000225 3.46607131362012e-09 441213.844717753 -590978.692496833;-0.00015 3.38053349329781e-09 457744.798197402 -578269.158062098;-7.5e-05 3.29229332622486e-09 473909.837489103 -565097.364110224]  x2=[-0.002325 1.36743129949518e-08 0 0;-0.00225 1.37602500095894e-08 0 0;-0.002175 1.38351872909083e-08 0 0;-0.0021 1.38990649351923e-08 0 0;-0.002025 1.39518318796298e-08 0 0;-0.00195 1.3993445943133e-08 0 0;-0.001875 1.40238738600562e-08 0 0;-0.0018 1.40430913067881e-08 0 0;-0.001725 1.40510829211958e-08 0 0;-0.00165 1.40478423149052e-08 0 0;-0.001575 1.40333720784072e-08 0 0;-0.0015 1.40076837789875e-08 0 0;-0.001425 1.39707979514796e-08 -189823.746323601 -705777.196573694;-0.00135 1.39227440818497e-08 -169795.146815445 -710861.533020316;-0.001275 1.38635605836259e-08 -149630.815664878 -715377.617633987;-0.0012 1.37932947671911e-08 -129346.871929697 -719321.840325766;-0.001125 1.37120028019639e-08 -108959.530284169 -722691.048144382;-0.00105 1.36197496714975e-08 -88485.0880572684 -725482.547796656;-0.000975 1.35166091215329e-08 -67939.9122048419 -727694.107800476;-0.0009 1.34026636010476e-08 -47340.4262261144 -729323.960268613;-0.000825 1.32780041963472e-08 -26703.0970349947 -730370.802321943;-0.00075 1.31427305582526e-08 -6044.42179667621 -730833.797130944;-0.000675 1.29969508224402e-08 14619.0852599438 -730712.574584651;-0.0006 1.28407815230003e-08 35270.9060434865 -730007.231586512;-0.000525 1.26743474992815e-08 55894.531804401 -728718.331976929;-0.00045 1.24977817960958e-08 76473.4763318061 -726846.906082527;-0.000375 1.23112255573648e-08 96991.2891323149 -724394.449892533;-0.0003 1.21148279132913e-08 117431.568580308 -721362.923862902;-0.000225 1.1908745861147e-08 137777.975029141 -717754.751349158;-0.00015 1.16931441397712e-08 158014.24387281 -713572.816669202;-7.5e-05 1.14681950978812e-08 178124.198547625 -708820.46279763]  x3=[-0.002325 3.2851098960138e-12 0 0;-0.00225 3.77872557180869e-12 0 0;-0.002175 4.26932059219791e-12 0 0;-0.0021 4.75650278302853e-12 0 0;-0.002025 5.23988269831133e-12 0 0;-0.00195 5.71907393153799e-12 0 0;-0.001875 6.19369342456854e-12 0 0;-0.0018 6.66336177384218e-12 0 0;-0.001725 7.12770353366667e-12 0 0;-0.00165 7.58634751634386e-12 0 0;-0.001575 8.0389270888915e-12 0 0;-0.0015 8.48508046612399e-12 0 0;-0.001425 8.92445099985794e-12 -163.959464484036 -404.071950170082;-0.00135 9.35668746401129e-12 -152.470711052459 -408.545860687759;-0.001275 9.78144433536802e-12 -140.860074867348 -412.693185895363;-0.0012 1.01983820697842e-11 -129.136837293619 -416.510610484579;-0.001125 1.06071673736142e-11 -117.310369708017 -419.995082864601;-0.00105 1.10074734701409e-11 -105.39012600778 -423.143817601521;-0.000975 1.13989803607956e-11 -93.3856350533348 -425.954297644967;-0.0009 1.178137508096e-11 -81.3064930510762 -428.424276340196;-0.000825 1.21543519501459e-11 -69.1623558823037 -430.551779224029;-0.00075 1.25176128163506e-11 -56.9629313844584 -432.335105603214;-0.000675 1.28708672943958e-11 -44.7179715908265 -433.772829913929;-0.0006 1.32138329980568e-11 -32.4372649349127 -434.863802861357;-0.000525 1.35462357657975e-11 -20.1306284257168 -435.607152338417;-0.00045 1.38678098799314e-11 -7.80789980016631 -436.002284122911;-0.000375 1.41782982790319e-11 4.52107034101956 -436.048882352535;-0.0003 1.44774527634234e-11 16.8464264077495 -435.746909777379;-0.000225 1.47650341935883e-11 29.1583156989681 -435.096607789698;-0.00015 1.50408126813314e-11 41.4468962787541 -434.098496230951;-7.5e-05 1.53045677735492e-11 53.7023448438137 -432.753372976247]  x4=[-0.002325 1.46293659959403e-11 0 0;-0.00225 1.45343490074241e-11 0 0;-0.002175 1.44277134826945e-11 0 0;-0.0021 1.43095446645581e-11 0 0;-0.002025 1.41799370153604e-11 0 0;-0.00195 1.40389941414728e-11 0 0;-0.001875 1.38868287104724e-11 0 0;-0.0018 1.37235623610764e-11 0 0;-0.001725 1.35493256059065e-11 0 0;-0.00165 1.33642577271589e-11 0 0;-0.001575 1.31685066652642e-11 0 0;-0.0015 1.29622289006262e-11 0 0;-0.001425 1.27455893285338e-11 -1447.81766818182 -4750.17763764077;-0.00135 1.25187611273462e-11 -1312.94851541782 -4789.20959204463;-0.001275 1.22819256200568e-11 -1177.02981169937 -4824.41312557796;-0.0012 1.20352721293466e-11 -1040.17020835862 -4855.76009707471;-0.001125 1.1778997826242e-11 -902.479108868437 -4883.22544824548;-0.00105 1.15133075724998e-11 -764.066581387022 -4906.78722370877;-0.000975 1.12384137568437e-11 -625.043270771056 -4926.42658854179;-0.0009 1.09545361251839e-11 -485.520310127919 -4942.12784333679;-0.000825 1.06619016049556e-11 -345.609231977576 -4953.87843675091;-0.00075 1.03607441237168e-11 -205.421879095188 -4961.66897553958;-0.000675 1.00513044221503e-11 -65.070315105711 -4965.49323206528;-0.0006 9.73382986161883e-12 75.3332650980515 -4965.34814927587;-0.000525 9.40857422642856e-12 215.676625042332 -4961.23384314829;-0.00045 9.0757975209577e-12 355.847576392518 -4953.15360259593;-0.000375 8.73576576181294e-12 495.734068634785 -4941.11388683945;-0.0003 8.38875076517989e-12 635.224278647571 -4925.1243202434;-0.000225 8.03502992953734e-12 774.206700091264 -4905.19768462268;-0.00015 7.6748860139092e-12 912.570232544664 -4881.34990902491;-7.5e-05 7.30860691183124e-12 1050.20427031696 -4853.60005699702]  x5=0.00231306500901259  V1=ones(3,3)  V2=ones(3,3)  I1=ones(3,3)  I2=ones(3,3)  nHarmo=1  Measurements=None  Decoupling=on  VsMag0=[602176.302414572 602177.107483061 602176.165720936]  VrMag0=[596743.737336323 596743.911083336 596743.706580344]  VsAngle0=[11.6043495452581 -108.395709698235 131.604253585468]  VrAngle0=[-14.273856882167 -134.273869923453 105.726122150021]  IsMag0=[359.486265157467 359.489496854362 359.491918798388]  IrMag0=[4093.84062560504 4093.84102057864 4093.83505039158]  IsAngle0=[-21.3064747486245 -141.305731641579 98.6934507450523]  IrAngle0=[-16.1707432095116 -136.170836500556 103.82920535766]
      settings: AttributesFormatString=\n  LibrarySourceBlock=sps_lib/Power Grid Elements/Distributed Parameters Line
  MIC-MAN 60 km : spsDistributedParametersLineLib/Distributed Parameters Line  Phases=3  Length=60  Frequency=60  Resistance="[0.01273  0.3864]"  Inductance="[0.9337e-3  4.1264e-3]"  Capacitance=[12.74e-9 7.751e-9]  x1=[-0.000375 3.8961833539361e-09 367056.472396769 -647795.562767882;-0.0003 3.80974254835898e-09 385223.31391595 -637159.785534291;-0.000225 3.72025629287972e-09 403082.213812101 -626014.672517016;-0.00015 3.62779612144176e-09 420618.895953895 -614369.132948876;-7.5e-05 3.53243594529146e-09 437819.341785948 -602232.476096019]  x2=[-0.000375 1.07742798642558e-09 381674.193271371 -619636.360457079;-0.0003 1.02648156742245e-09 399039.114850727 -608598.586309068;-0.000225 9.7471459476002e-10 416085.050667174 -597074.307763032;-0.00015 9.2216845016417e-10 432798.374460433 -585072.737150913;-7.5e-05 8.68885138218909e-10 449165.725855185 -572603.468344629]  x3=[-0.000375 -8.62333115106169e-12 2615.73591803649 -3083.53120523823;-0.0003 -9.4214304465362e-12 2701.86358792154 -3008.35057124431;-0.000225 -1.02119983946645e-11 2785.8314293943 -2930.76510783305;-0.00015 -1.09944030275249e-11 2867.57231984706 -2850.83683563679;-7.5e-05 -1.17680189028251e-11 2947.02091686265 -2768.6296480934]  x4=[-0.000375 2.42768153167114e-11 -38.3285845653421 -1696.07516225673;-0.0003 2.49227530370171e-11 9.6357897044698 -1696.48092157495;-0.000225 2.55487678898759e-11 57.5924612714245 -1695.53054000149;-0.00015 2.61543594485928e-11 105.503094306033 -1693.22477725684;-7.5e-05 2.67390436125417e-11 153.329389781305 -1689.56547653246]  x5=0.000339324940197445  V1=ones(3,3)  V2=ones(3,3)  I1=ones(3,3)  I2=ones(3,3)  nHarmo=1  Measurements=None  Decoupling=on  VsMag0=[607930.23167611 607930.976808519 607930.152146887]  VrMag0=[594207.380493472 594208.10130569 594207.286862311]  VsAngle0=[7.63692875074935 -112.363120449623 127.636843332422]  VrAngle0=[9.73160889879769 -110.268441654031 129.731523430554]  IsMag0=[3306.19691878135 3306.20035207237 3306.19654855249]  IrMag0=[1387.14843174292 1387.15088256342 1387.14865267779]  IsAngle0=[18.4076953761299 -101.592346383785 138.40762296912]  IrAngle0=[-23.1945765462506 -143.194624454317 96.8053118315588]
      settings: AttributesFormatString=\n  LibrarySourceBlock=sps_lib/Power Grid Elements/Distributed Parameters Line
  Regulateurs6 : Subsystem
  Regulateurs7 : Subsystem
  "MIC7a " : PMIOPort  Side=Left
  MIC7b : PMIOPort  Port=2  Side=Left
  MIC7c : PMIOPort  Port=3  Side=Left
  QUE7a : PMIOPort  Port=4  Side=Left
  QUE7b : PMIOPort  Port=5  Side=Left
  QUE7c : PMIOPort  Port=6  Side=Left
  wires:
  Regulateurs6/1(Pm) -> "B_6 CHU-5600 MVA "/1
  Regulateurs6/2(Vf) -> "B_6 CHU-5600 MVA "/2
  "B_6 CHU-5600 MVA "/1 -> Regulateurs6/1(m)
  Regulateurs7/1(Pm) -> B_7 MAN 5000 MVA/1
  Regulateurs7/2(Vf) -> B_7 MAN 5000 MVA/2
  B_7 MAN 5000 MVA/1 -> Regulateurs7/1(m)
  connections:
  "Cs PER "/RConn3 -- MIC-LTD 409 km/LConn3
  "Cs PER "/RConn2 -- MIC-LTD 409 km/LConn2
  "Cs PER "/RConn1 -- MIC-LTD 409 km/LConn1
  Cs BER/RConn3 -- MAN-LEV 3*379km/LConn3
  Cs BER/RConn2 -- MAN-LEV 3*379km/LConn2
  Cs BER/RConn1 -- MAN-LEV 3*379km/LConn1
  Cs ARNS2/RConn3 -- ARN-MAN 2*169km/LConn3
  Cs ARNS2/RConn2 -- ARN-MAN 2*169km/LConn2
  Cs ARNS2/RConn1 -- ARN-MAN 2*169km/LConn1
  CHU-ARN 3*450km/RConn3 -- "Cs MTG+ARNN "/LConn3
  CHU-ARN 3*450km/RConn2 -- "Cs MTG+ARNN "/LConn2
  CHU-ARN 3*450km/RConn1 -- "Cs MTG+ARNN "/LConn1
  Load Flow Bus2/LConn1 -- 5600 MVA 13.8 kV/735 kV1/RConn3 -- CHU-ARN 3*450km/LConn3 -- CHU 330 Mvar/LConn3
  5600 MVA 13.8 kV/735 kV1/RConn2 -- CHU-ARN 3*450km/LConn2 -- CHU 330 Mvar/LConn2
  5600 MVA 13.8 kV/735 kV1/RConn1 -- CHU-ARN 3*450km/LConn1 -- CHU 330 Mvar/LConn1
  "B_6 CHU-5600 MVA "/RConn3 -- Load Flow Bus1/LConn1 -- 5600 MVA 13.8 kV/735 kV1/LConn3 -- 280 MW/LConn3
  5600 MVA 13.8 kV/735 kV1/LConn2 -- "B_6 CHU-5600 MVA "/RConn2 -- 280 MW/LConn2
  5600 MVA 13.8 kV/735 kV1/LConn1 -- "B_6 CHU-5600 MVA "/RConn1 -- 280 MW/LConn1
  "Cs ARNS1 "/RConn1 -- ARN-MIC 180km/LConn1
  "Cs ARNS1 "/RConn2 -- ARN-MIC 180km/LConn2
  "Cs ARNS1 "/RConn3 -- ARN-MIC 180km/LConn3
  "Cs PER "/LConn3 -- Load Flow Bus6/LConn1 -- MIC7c/RConn1 -- MIC-MAN 60 km/LConn3 -- ARN-MIC 180km/RConn3
  "Cs PER "/LConn2 -- MIC7b/RConn1 -- ARN-MIC 180km/RConn2 -- MIC-MAN 60 km/LConn2
  "Cs PER "/LConn1 -- "MIC7a "/RConn1 -- ARN-MIC 180km/RConn1 -- MIC-MAN 60 km/LConn1
  ARN-MAN 2*169km/RConn1 -- MAN7/LConn1
  ARN-MAN 2*169km/RConn2 -- MAN7/LConn2
  ARN-MAN 2*169km/RConn3 -- MAN7/LConn3
  Cs BER/LConn1 -- 5000 MVA 13.8 kV/735 kV2/RConn1 -- MIC-MAN 60 km/RConn1 -- MAN-MIC 1650 Mvar/LConn1 -- MAN7/RConn1
  Cs BER/LConn2 -- 5000 MVA 13.8 kV/735 kV2/RConn2 -- MIC-MAN 60 km/RConn2 -- MAN-MIC 1650 Mvar/LConn2 -- MAN7/RConn2
  Cs BER/LConn3 -- Load Flow Bus5/LConn1 -- 5000 MVA 13.8 kV/735 kV2/RConn3 -- MIC-MAN 60 km/RConn3 -- MAN-MIC 1650 Mvar/LConn3 -- MAN7/RConn3
  B_7 MAN 5000 MVA/RConn1 -- 5000 MVA 13.8 kV/735 kV2/LConn1 -- 250 MW/LConn1
  B_7 MAN 5000 MVA/RConn2 -- 5000 MVA 13.8 kV/735 kV2/LConn2 -- 250 MW/LConn2
  B_7 MAN 5000 MVA/RConn3 -- 5000 MVA 13.8 kV/735 kV2/LConn3 -- Load Flow Bus3/LConn1 -- 250 MW/LConn3
  MIC-LTD 409 km/RConn2 -- MAN-LEV 3*379km/RConn2 -- QUE7b/RConn1
  Cs ARNS2/LConn1 -- ARN 990 Mvar/LConn1 -- "Cs MTG+ARNN "/RConn1 -- "Cs ARNS1 "/LConn1
  Cs ARNS2/LConn2 -- ARN 990 Mvar/LConn2 -- "Cs MTG+ARNN "/RConn2 -- "Cs ARNS1 "/LConn2
  Cs ARNS2/LConn3 -- Load Flow Bus4/LConn1 -- "Cs ARNS1 "/LConn3 -- ARN 990 Mvar/LConn3 -- "Cs MTG+ARNN "/RConn3
  MIC-LTD 409 km/RConn1 -- QUE7a/RConn1 -- MAN-LEV 3*379km/RConn1
  MIC-LTD 409 km/RConn3 -- QUE7c/RConn1 -- MAN-LEV 3*379km/RConn3
